simulink library "BEML_EMU_PneumaticsInput_Lib"  (R2019b)
settings: Solver=VariableStepAuto  StartTime=0.0  StopTime=10.0  RelTol=1e-3
undefined symbols (not defined in the file): AuxiliaryCompressorOn, BogieControl, BogieSupportedMasses, ElectricalSignals, HornHighControl, HornLowControl, InputControlStates, MainCompressorOn, NoEmergencyBrakeValve, PantographRaiseValve, ParkingBrakeApplyCmd, ParkingBrakeReleaseCmd, PhysicalSignals, PneumaticallyCoupled, PneumaticsSampleTime, RemoteHornIsolate, RemoteMagnetValve1, RemoteMagnetValve2, Reset, StartupState, TCMSBrakingDemand, VCBCloseCmd
libraries: VectorOperationsLib x1
settings Model: Creator=rleighton  LastModifiedBy=hinganes
settings DebuggingCC: ArithmeticOperatorsInVariantConditions=warning
settings SFSimCC: SimUseLocalCustomCode=off  CustomCodeUndefinedFunction=UseInterfaceOnly
settings RTWCC: RTWUseLocalCustomCode=off
settings CodeAppCC: StateflowObjectComments=on

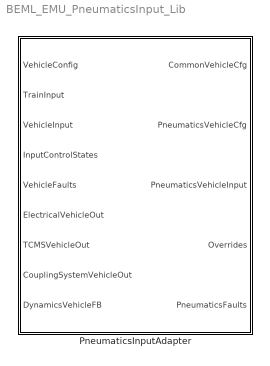
== system BEML_EMU_PneumaticsInput_Lib ==
  PneumaticsInputAdapter : Subsystem  TreatAsAtomicUnit=on  SystemSampleTime=PneumaticsSampleTime

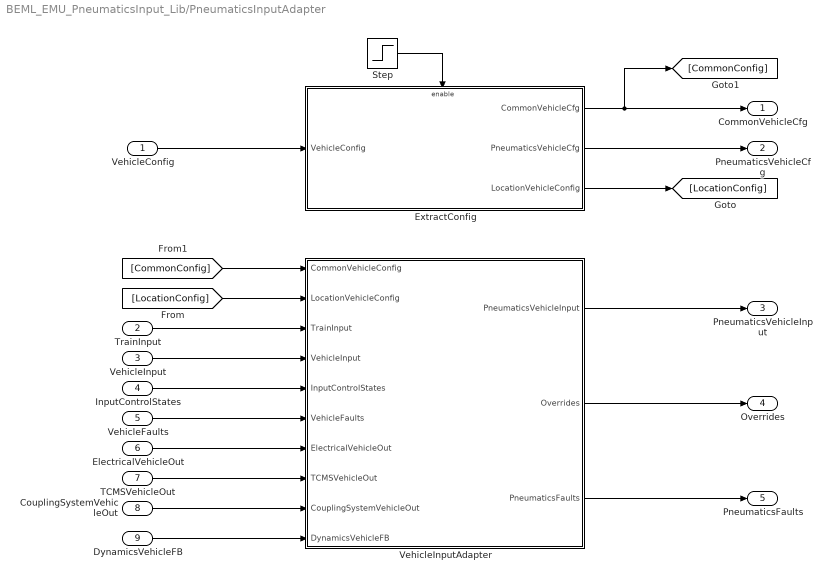
== system BEML_EMU_PneumaticsInput_Lib/PneumaticsInputAdapter ==
  VehicleConfig : Inport
  TrainInput : Inport  Port=2
  VehicleInput : Inport  Port=3
  InputControlStates : Inport  Port=4
  VehicleFaults : Inport  Port=5
  ElectricalVehicleOut : Inport  Port=6
  TCMSVehicleOut : Inport  Port=7
  CouplingSystemVehicleOut : Inport  Port=8
  DynamicsVehicleFB : Inport  Port=9
  ExtractConfig : Subsystem
  Step : Step  Before=1  After=0
  VehicleInputAdapter : Subsystem
  CommonVehicleCfg : Outport  VectorParamsAs1DForOutWhenUnconnected=off
  PneumaticsVehicleCfg : Outport  Port=2  VectorParamsAs1DForOutWhenUnconnected=off
  PneumaticsVehicleInput : Outport  Port=3  VectorParamsAs1DForOutWhenUnconnected=off
  Overrides : Outport  Port=4  VectorParamsAs1DForOutWhenUnconnected=off
  PneumaticsFaults : Outport  Port=5  VectorParamsAs1DForOutWhenUnconnected=off
  wires:
  TCMSVehicleOut/1 -> VehicleInputAdapter/8(TCMSVehicleOut)
  [CommonConfig] -> VehicleInputAdapter/1(CommonVehicleConfig)
  InputControlStates/1 -> VehicleInputAdapter/5(InputControlStates)
  [LocationConfig] -> VehicleInputAdapter/2(LocationVehicleConfig)
  ExtractConfig/3(LocationVehicleConfig) -> [LocationConfig]
  CouplingSystemVehicleOut/1 -> VehicleInputAdapter/9(CouplingSystemVehicleOut)
  VehicleInputAdapter/3(PneumaticsFaults) -> PneumaticsFaults/1
  VehicleInputAdapter/2(Overrides) -> Overrides/1
  VehicleInputAdapter/1(PneumaticsVehicleInput) -> PneumaticsVehicleInput/1
  VehicleFaults/1 -> VehicleInputAdapter/6(VehicleFaults)
  Step/1 -> ExtractConfig/Enable
  ExtractConfig/2(PneumaticsVehicleCfg) -> PneumaticsVehicleCfg/1
  ExtractConfig/1(CommonVehicleCfg) -> CommonVehicleCfg/1, [CommonConfig]
  VehicleConfig/1 -> ExtractConfig/1(VehicleConfig)
  DynamicsVehicleFB/1 -> VehicleInputAdapter/10(DynamicsVehicleFB)
  ElectricalVehicleOut/1 -> VehicleInputAdapter/7(ElectricalVehicleOut)
  VehicleInput/1 -> VehicleInputAdapter/4(VehicleInput)
  TrainInput/1 -> VehicleInputAdapter/3(TrainInput)

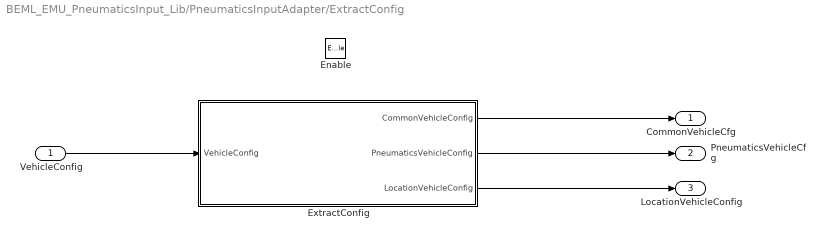
== system BEML_EMU_PneumaticsInput_Lib/PneumaticsInputAdapter/ExtractConfig ==
  VehicleConfig : Inport
  Enable : EnablePort
  ExtractConfig : Subsystem
  CommonVehicleCfg : Outport  VectorParamsAs1DForOutWhenUnconnected=off
  PneumaticsVehicleCfg : Outport  Port=2  VectorParamsAs1DForOutWhenUnconnected=off
  LocationVehicleConfig : Outport  Port=3  VectorParamsAs1DForOutWhenUnconnected=off
  wires:
  ExtractConfig/3(LocationVehicleConfig) -> LocationVehicleConfig/1
  VehicleConfig/1 -> ExtractConfig/1(VehicleConfig)
  ExtractConfig/1(CommonVehicleConfig) -> CommonVehicleCfg/1
  ExtractConfig/2(PneumaticsVehicleConfig) -> PneumaticsVehicleCfg/1

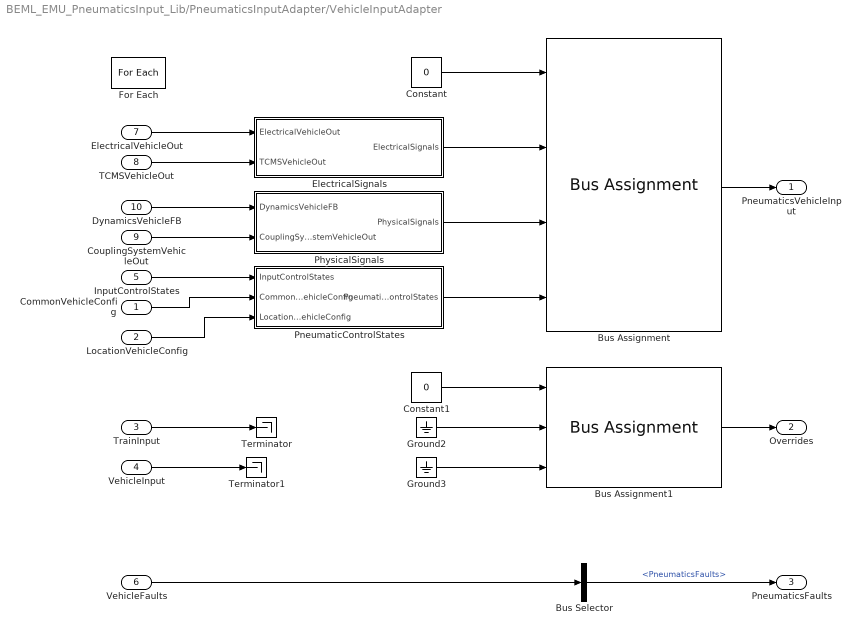
== system BEML_EMU_PneumaticsInput_Lib/PneumaticsInputAdapter/VehicleInputAdapter ==
  CommonVehicleConfig : Inport  Partition=on  PartitionDimension=1  PartitionWidth=1  PartitionOffset=0
  LocationVehicleConfig : Inport  Port=2  Partition=on  PartitionDimension=1  PartitionWidth=1  PartitionOffset=0
  TrainInput : Inport  Port=3
  VehicleInput : Inport  Port=4  Partition=on  PartitionDimension=1  PartitionWidth=1  PartitionOffset=0
  InputControlStates : Inport  Port=5  Partition=on  PartitionDimension=1  PartitionWidth=1  PartitionOffset=0
  VehicleFaults : Inport  Port=6  Partition=on  PartitionDimension=1  PartitionWidth=1  PartitionOffset=0
  ElectricalVehicleOut : Inport  Port=7  Partition=on  PartitionDimension=1  PartitionWidth=1  PartitionOffset=0
  TCMSVehicleOut : Inport  Port=8  Partition=on  PartitionDimension=1  PartitionWidth=1  PartitionOffset=0
  CouplingSystemVehicleOut : Inport  Port=9  Partition=on  PartitionDimension=1  PartitionWidth=1  PartitionOffset=0
  DynamicsVehicleFB : Inport  Port=10  Partition=on  PartitionDimension=1  PartitionWidth=1  PartitionOffset=0
  Bus Assignment : BusAssignment  AssignedSignals=ElectricalSignals,PhysicalSignals,InputControlStates
  Bus Assignment1 : BusAssignment  AssignedSignals=Reset,StartupState
  Bus Selector : BusSelector  OutputSignals=PneumaticsFaults
  Constant : Constant  Value=0  OutDataTypeStr=Bus: BD_PneumaticsSystem_In_Vehicle
  Constant1 : Constant  Value=0  OutDataTypeStr=Bus: BD_PneumaticsSystem_In_Overrides
  ElectricalSignals : Subsystem
  For Each : ForEach  DisableCoverage=on
  Ground2 : Ground
  Ground3 : Ground
  PhysicalSignals : Subsystem
  PneumaticControlStates : Subsystem
  Terminator : Terminator
  Terminator1 : Terminator
  PneumaticsVehicleInput : Outport  ConcatenationDimension=1  VectorParamsAs1DForOutWhenUnconnected=off
  Overrides : Outport  Port=2  ConcatenationDimension=1  VectorParamsAs1DForOutWhenUnconnected=off
  PneumaticsFaults : Outport  Port=3  ConcatenationDimension=1  VectorParamsAs1DForOutWhenUnconnected=off
  wires:
  TCMSVehicleOut/1 -> ElectricalSignals/2(TCMSVehicleOut)
  CommonVehicleConfig/1 -> PneumaticControlStates/2(CommonVehicleConfig)
  PneumaticControlStates/1(PneumaticControlStates) -> Bus Assignment/4
  InputControlStates/1 -> PneumaticControlStates/1(InputControlStates)
  LocationVehicleConfig/1 -> PneumaticControlStates/3(LocationVehicleConfig)
  CouplingSystemVehicleOut/1 -> PhysicalSignals/2(CouplingSystemVehicleOut)
  PhysicalSignals/1(PhysicalSignals) -> Bus Assignment/3
  ElectricalSignals/1(ElectricalSignals) -> Bus Assignment/2
  ElectricalVehicleOut/1 -> ElectricalSignals/1(ElectricalVehicleOut)
  Bus Selector/1 -> PneumaticsFaults/1  "<PneumaticsFaults>"
  Bus Assignment1/1 -> Overrides/1
  Ground2/1 -> Bus Assignment1/2
  Ground3/1 -> Bus Assignment1/3
  Constant1/1 -> Bus Assignment1/1
  Bus Assignment/1 -> PneumaticsVehicleInput/1
  Constant/1 -> Bus Assignment/1
  DynamicsVehicleFB/1 -> PhysicalSignals/1(DynamicsVehicleFB)
  VehicleFaults/1 -> Bus Selector/1
  VehicleInput/1 -> Terminator1/1
  TrainInput/1 -> Terminator/1

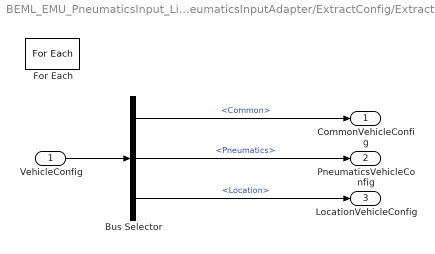
== system BEML_EMU_PneumaticsInput_Lib/PneumaticsInputAdapter/ExtractConfig/ExtractConfig ==
  VehicleConfig : Inport  Partition=on  PartitionDimension=1  PartitionWidth=1  PartitionOffset=0  BusOutputAsStruct=on
  Bus Selector : BusSelector  OutputSignals=Common,Pneumatics,Location
  For Each : ForEach  DisableCoverage=on
  CommonVehicleConfig : Outport  ConcatenationDimension=1  VectorParamsAs1DForOutWhenUnconnected=off
  PneumaticsVehicleConfig : Outport  Port=2  ConcatenationDimension=1  VectorParamsAs1DForOutWhenUnconnected=off
  LocationVehicleConfig : Outport  Port=3  ConcatenationDimension=1  VectorParamsAs1DForOutWhenUnconnected=off
  wires:
  Bus Selector/3 -> LocationVehicleConfig/1  "<Location>"
  Bus Selector/2 -> PneumaticsVehicleConfig/1  "<Pneumatics>"
  Bus Selector/1 -> CommonVehicleConfig/1  "<Common>"
  VehicleConfig/1 -> Bus Selector/1

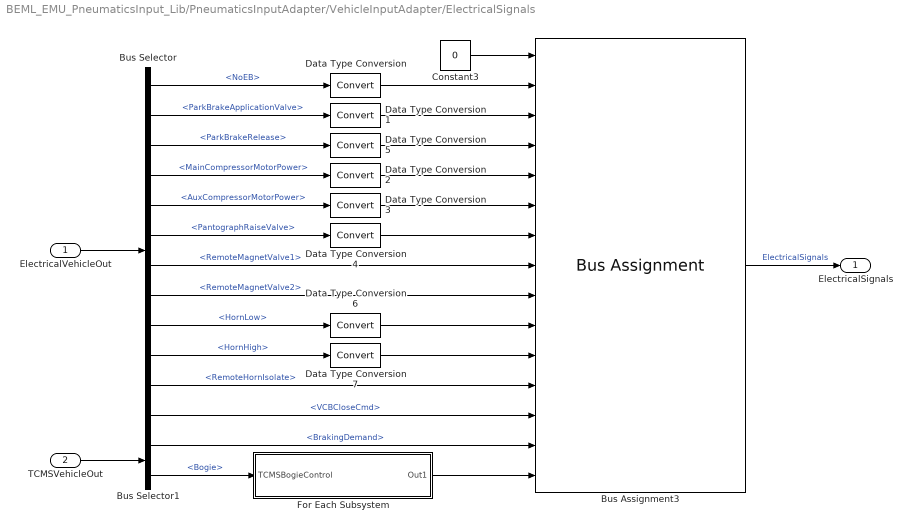
== system BEML_EMU_PneumaticsInput_Lib/PneumaticsInputAdapter/VehicleInputAdapter/ElectricalSignals ==
  ElectricalVehicleOut : Inport
  TCMSVehicleOut : Inport  Port=2
  Bus Assignment3 : BusAssignment  AssignedSignals=NoEmergencyBrakeValve,ParkingBrakeApplyCmd,ParkingBrakeReleaseCmd,MainCompressorOn,AuxiliaryCompressorOn,PantographRaiseValve,RemoteMagnetValve1,RemoteMagnetValve2,HornLowControl,HornHighControl,RemoteHornIsolate,VCBCloseCmd,TCMSBrakingDemand,BogieControl
  Bus Selector : BusSelector  OutputSignals=Braking.NoEB,Pneumatics.ParkBrakeApplicationValve,Pneumatics.ParkBrakeRelease,Pneumatics.MainCompressorMotorPower,Pneumatics.AuxCompressorMotorPower,Pneumatics.PantographRaiseValve,Pneumatics.RemoteMagnetValve1,Pneumatics.RemoteMagnetValve2,Pneumatics.HornLow,Pneumatics.HornHigh,Pneumatics.RemoteHornIsolate,Pneumatics.VCBCloseCmd
  Bus Selector1 : BusSelector  OutputSignals=Control.PneumaticSystem.BrakingDemand,Control.TractionSBraking.Bogie
  Constant3 : Constant  Value=0  OutDataTypeStr=Bus: BD_PneumaticsSystem_In_Vehicle_ElectricalSignals
  Data Type Conversion{,1..7} (8 alike) : DataTypeConversion
  For Each Subsystem : Subsystem  TreatAsAtomicUnit=on
  ElectricalSignals : Outport
  wires:
  Bus Selector1/1 -> Bus Assignment3/14  "<BrakingDemand>"
  Bus Selector/12 -> Bus Assignment3/13  "<VCBCloseCmd>"
  Data Type Conversion7/1 -> Bus Assignment3/11
  Bus Selector/10 -> Data Type Conversion7/1  "<HornHigh>"
  Data Type Conversion6/1 -> Bus Assignment3/10
  Bus Selector/11 -> Bus Assignment3/12  "<RemoteHornIsolate>"
  Bus Selector/9 -> Data Type Conversion6/1  "<HornLow>"
  Bus Selector/7 -> Bus Assignment3/8  "<RemoteMagnetValve1>"
  Bus Selector/8 -> Bus Assignment3/9  "<RemoteMagnetValve2>"
  Data Type Conversion5/1 -> Bus Assignment3/4
  Bus Selector/3 -> Data Type Conversion5/1  "<ParkBrakeRelease>"
  For Each Subsystem/1(Out1) -> Bus Assignment3/15
  Bus Selector1/2 -> For Each Subsystem/1(TCMSBogieControl)  "<Bogie>"
  Data Type Conversion4/1 -> Bus Assignment3/7
  Data Type Conversion3/1 -> Bus Assignment3/6
  Data Type Conversion2/1 -> Bus Assignment3/5
  Data Type Conversion1/1 -> Bus Assignment3/3
  Data Type Conversion/1 -> Bus Assignment3/2
  TCMSVehicleOut/1 -> Bus Selector1/1
  Bus Selector/1 -> Data Type Conversion/1  "<NoEB>"
  Bus Selector/2 -> Data Type Conversion1/1  "<ParkBrakeApplicationValve>"
  Bus Selector/6 -> Data Type Conversion4/1  "<PantographRaiseValve>"
  Bus Selector/4 -> Data Type Conversion2/1  "<MainCompressorMotorPower>"
  Bus Selector/5 -> Data Type Conversion3/1  "<AuxCompressorMotorPower>"
  Constant3/1 -> Bus Assignment3/1
  Bus Assignment3/1 -> ElectricalSignals/1  "ElectricalSignals"
  ElectricalVehicleOut/1 -> Bus Selector/1

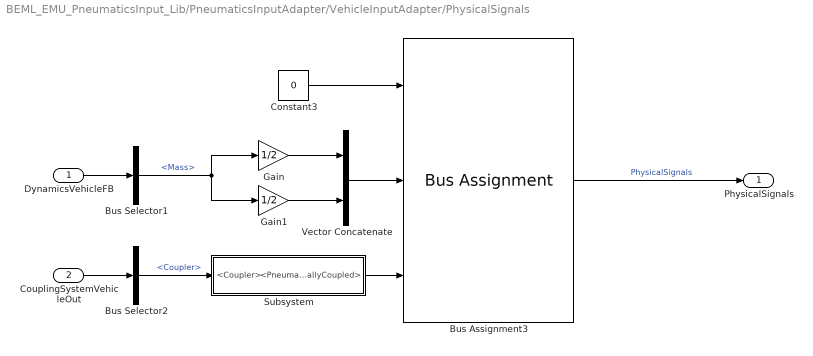
== system BEML_EMU_PneumaticsInput_Lib/PneumaticsInputAdapter/VehicleInputAdapter/PhysicalSignals ==
  DynamicsVehicleFB : Inport
  CouplingSystemVehicleOut : Inport  Port=2
  Bus Assignment3 : BusAssignment  AssignedSignals=BogieSupportedMasses,PneumaticallyCoupled
  Bus Selector1 : BusSelector  OutputSignals=Inertia.Mass
  Bus Selector2 : BusSelector  OutputSignals=Couplers.Coupler
  Constant3 : Constant  Value=0  OutDataTypeStr=Bus: BD_PneumaticsSystem_In_Vehicle_PhysicalSignals
  Gain : Gain  Gain=1/2
  Gain1 : Gain  Gain=1/2
  Subsystem : Subsystem
  Vector Concatenate : Concatenate
  PhysicalSignals : Outport
  wires:
  Bus Selector2/1 -> Subsystem/1(<Coupler>)  "<Coupler>"
  Subsystem/1(<PneumaticallyCoupled>) -> Bus Assignment3/3
  CouplingSystemVehicleOut/1 -> Bus Selector2/1
  Gain1/1 -> Vector Concatenate/2
  Gain/1 -> Vector Concatenate/1
  Bus Selector1/1 -> Gain/1, Gain1/1  "<Mass>"
  Vector Concatenate/1 -> Bus Assignment3/2
  DynamicsVehicleFB/1 -> Bus Selector1/1
  Bus Assignment3/1 -> PhysicalSignals/1  "PhysicalSignals"
  Constant3/1 -> Bus Assignment3/1

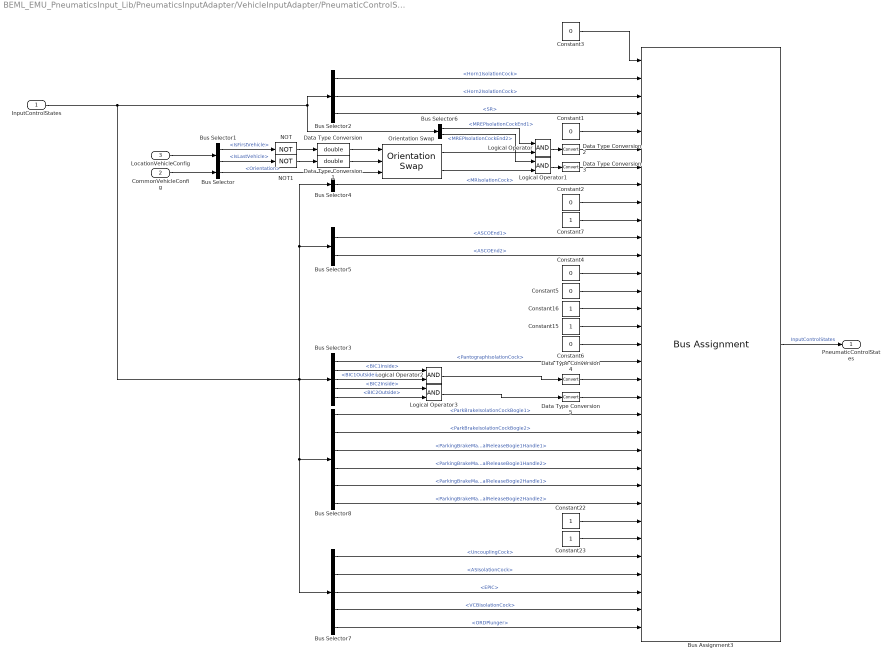
== system BEML_EMU_PneumaticsInput_Lib/PneumaticsInputAdapter/VehicleInputAdapter/PneumaticControlStates ==
  InputControlStates : Inport
  CommonVehicleConfig : Inport  Port=2
  LocationVehicleConfig : Inport  Port=3
  Bus Assignment3 : BusAssignment  AssignedSignals=HornLowIsolationCock,HornHighIsolationCock,BrakeSupplyReservoirIsolationCock,BrakeSupplyReservoirDrainCock,InterCarIsolationCockEnd1,InterCarIsolationCockEnd2,MainReservoirIsolationCock,MainReservoirDrainCock,MainAirSupplyIsolationCock,AirSuspensionSystemIsolationCockBogie1,AirSuspensionSystemIsolationCockBogie2,AirSuspensionSystemDrainCockBogie1,AirSuspensionSystemDrainCockBogie2,AuxiliaryCompressorIsolationCock,AuxiliaryReservoirIsolationCock,AuxiliaryReservoirDrainCock,PantographAirSupplyIsolationCock,BrakeCylinderIsolationCockBogie1,BrakeCylinderIsolationCockBogie2,ParkingBrakeIsolationCockBogie1,ParkingBrakeIsolationCockBogie2,ParkingBrakeManualReleaseBogie1Handle1,ParkingBrakeManualReleaseBogie1Handle2,ParkingBrakeManualReleaseBogie2Handle1,ParkingBrakeManualReleaseBogie2Handle2,SandingSystemIsolationCockBogie1,SandingSystemIsolationCockBogie2,UncouplingIsolationCock,AirSuspensionReservoirIsolationCock,EPIsolationCock,VCBIsolationCock,ORDPlunger
  Bus Selector : BusSelector  OutputSignals=Orientation
  Bus Selector1 : BusSelector  OutputSignals=IsFirstVehicle,IsLastVehicle
  Bus Selector2 : BusSelector  OutputSignals=Horn1IsolationCock,Horn2IsolationCock,SR
  Bus Selector3 : BusSelector  OutputSignals=PantographIsolationCock,BIC1Inside,BIC1Outside,BIC2Inside,BIC2Outside
  Bus Selector4 : BusSelector  OutputSignals=MRIsolationCock
  Bus Selector5 : BusSelector  OutputSignals=ASCOEnd1,ASCOEnd2
  Bus Selector6 : BusSelector  OutputSignals=MREPIsolationCockEnd1,MREPIsolationCockEnd2
  Bus Selector7 : BusSelector  OutputSignals=UncouplingCock,ASIsolationCock,EPIC,VCBIsolationCock,ORDPlunger
  Bus Selector8 : BusSelector  OutputSignals=ParkBrakeIsolationCockBogie1,ParkBrakeIsolationCockBogie2,ParkingBrakeManualReleaseBogie1Handle1,ParkingBrakeManualReleaseBogie1Handle2,ParkingBrakeManualReleaseBogie2Handle1,ParkingBrakeManualReleaseBogie2Handle2
  Constant{1..2,4..6} (5 alike) : Constant  Value=0
  Constant{7,15..16,22..23} (5 alike) : Constant
  Constant3 : Constant  Value=0  OutDataTypeStr=Bus: BD_PneumaticsSystem_In_Vehicle_InputControlStates
  Data Type Conversion : DataTypeConversion  OutDataTypeStr=double
  Data Type Conversion1 : DataTypeConversion  OutDataTypeStr=double
  Data Type Conversion{2..5} (4 alike) : DataTypeConversion
  Logical Operator{,1..3} (4 alike) : Logic  AllPortsSameDT=off  OutDataTypeStr=boolean
  NOT : Logic  Operator=NOT  AllPortsSameDT=off  OutDataTypeStr=boolean
  NOT1 : Logic  Operator=NOT  AllPortsSameDT=off  OutDataTypeStr=boolean
  Orientation Swap : VectorOperationsLib/Orientation Swap
      settings: SourceProductName=Sydac Utilities
  PneumaticControlStates : Outport
  wires:
  Data Type Conversion5/1 -> Bus Assignment3/20
  Logical Operator3/1 -> Data Type Conversion5/1
  Bus Selector3/4 -> Logical Operator3/1  "<BIC2Inside>"
  Bus Selector3/5 -> Logical Operator3/2  "<BIC2Outside>"
  Data Type Conversion4/1 -> Bus Assignment3/19
  Logical Operator2/1 -> Data Type Conversion4/1
  Bus Selector3/3 -> Logical Operator2/2  "<BIC1Outside>"
  Bus Selector3/2 -> Logical Operator2/1  "<BIC1Inside>"
  Bus Selector7/5 -> Bus Assignment3/33  "<ORDPlunger>"
  Bus Selector7/4 -> Bus Assignment3/32  "<VCBIsolationCock>"
  Bus Selector7/3 -> Bus Assignment3/31  "<EPIC>"
  Constant7/1 -> Bus Assignment3/10
  Bus Selector7/2 -> Bus Assignment3/30  "<ASIsolationCock>"
  Bus Selector2/2 -> Bus Assignment3/3  "<Horn2IsolationCock>"
  CommonVehicleConfig/1 -> Bus Selector/1
  NOT/1 -> Data Type Conversion/1
  Orientation Swap/2 -> Logical Operator1/2
  Orientation Swap/1 -> Logical Operator/2
  Bus Selector1/2 -> NOT1/1  "<IsLastVehicle>"
  LocationVehicleConfig/1 -> Bus Selector1/1
  Data Type Conversion3/1 -> Bus Assignment3/7
  NOT1/1 -> Data Type Conversion1/1
  Logical Operator1/1 -> Data Type Conversion3/1
  Data Type Conversion1/1 -> Orientation Swap/2
  Constant2/1 -> Bus Assignment3/9
  Bus Selector2/3 -> Bus Assignment3/4  "<SR>"
  Bus Selector8/1 -> Bus Assignment3/21  "<ParkBrakeIsolationCockBogie1>"
  Constant6/1 -> Bus Assignment3/17
  Logical Operator/1 -> Data Type Conversion2/1
  InputControlStates/1 -> Bus Selector2/1, Bus Selector6/1, Bus Selector8/1, Bus Selector7/1, Bus Selector3/1, Bus Selector5/1, Bus Selector4/1
  Constant1/1 -> Bus Assignment3/5
  Constant5/1 -> Bus Assignment3/14
  Data Type Conversion2/1 -> Bus Assignment3/6
  Data Type Conversion/1 -> Orientation Swap/1
  Bus Selector2/1 -> Bus Assignment3/2  "<Horn1IsolationCock>"
  Bus Selector8/2 -> Bus Assignment3/22  "<ParkBrakeIsolationCockBogie2>"
  Constant15/1 -> Bus Assignment3/16
  Bus Selector5/2 -> Bus Assignment3/12  "<ASCOEnd2>"
  Bus Selector1/1 -> NOT/1  "<IsFirstVehicle>"
  Bus Selector3/1 -> Bus Assignment3/18  "<PantographIsolationCock>"
  Constant4/1 -> Bus Assignment3/13
  Bus Selector5/1 -> Bus Assignment3/11  "<ASCOEnd1>"
  Constant16/1 -> Bus Assignment3/15
  Bus Selector8/4 -> Bus Assignment3/24  "<ParkingBrakeManualReleaseBogie1Handle2>"
  Bus Selector8/5 -> Bus Assignment3/25  "<ParkingBrakeManualReleaseBogie2Handle1>"
  Bus Selector/1 -> Orientation Swap/3  "<Orientation>"
  Bus Selector6/2 -> Logical Operator1/1  "<MREPIsolationCockEnd2>"
  Bus Selector8/3 -> Bus Assignment3/23  "<ParkingBrakeManualReleaseBogie1Handle1>"
  Constant23/1 -> Bus Assignment3/28
  Constant22/1 -> Bus Assignment3/27
  Bus Selector4/1 -> Bus Assignment3/8  "<MRIsolationCock>"
  Bus Selector8/6 -> Bus Assignment3/26  "<ParkingBrakeManualReleaseBogie2Handle2>"
  Bus Selector7/1 -> Bus Assignment3/29  "<UncouplingCock>"
  Bus Selector6/1 -> Logical Operator/1  "<MREPIsolationCockEnd1>"
  Bus Assignment3/1 -> PneumaticControlStates/1  "InputControlStates"
  Constant3/1 -> Bus Assignment3/1

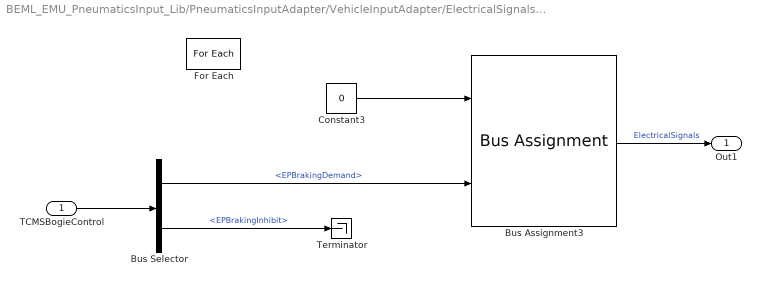
== system BEML_EMU_PneumaticsInput_Lib/PneumaticsInputAdapter/VehicleInputAdapter/ElectricalSignals/For Each Subsystem ==
  TCMSBogieControl : Inport  Partition=on  PartitionDimension=1  PartitionWidth=1  PartitionOffset=0
  Bus Assignment3 : BusAssignment  AssignedSignals=EPBrakingDemand
  Bus Selector : BusSelector  OutputSignals=EPBrakingDemand,EPBrakingInhibit
  Constant3 : Constant  Value=0  OutDataTypeStr=Bus: BD_PneumaticsSystem_In_Vehicle_ElectricalSignals_Bogie
  For Each : ForEach  DisableCoverage=on
  Terminator : Terminator
  Out1 : Outport  ConcatenationDimension=1
  wires:
  Bus Selector/2 -> Terminator/1  "<EPBrakingInhibit>"
  Bus Selector/1 -> Bus Assignment3/2  "<EPBrakingDemand>"
  TCMSBogieControl/1 -> Bus Selector/1
  Bus Assignment3/1 -> Out1/1  "ElectricalSignals"
  Constant3/1 -> Bus Assignment3/1

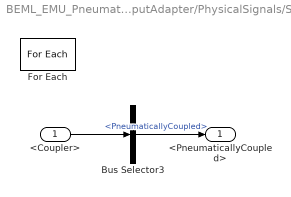
== system BEML_EMU_PneumaticsInput_Lib/PneumaticsInputAdapter/VehicleInputAdapter/PhysicalSignals/Subsystem ==
  <Coupler> : Inport  Partition=on  PartitionDimension=1  PartitionWidth=1  PartitionOffset=0
  Bus Selector3 : BusSelector  OutputSignals=CouplingInterface.PneumaticallyCoupled
  For Each : ForEach  DisableCoverage=on
  <PneumaticallyCoupled> : Outport  ConcatenationDimension=1
  wires:
  <Coupler>/1 -> Bus Selector3/1
  Bus Selector3/1 -> <PneumaticallyCoupled>/1  "<PneumaticallyCoupled>"
